simulink model "a20210929KillSwitchCharging"  (R2021b)
settings: Solver=VariableStepAuto  StartTime=0.0  StopTime=inf  RelTol=1e-3
model workspace (MAT data in the model file):
  Ah_chg = [23.2 23.2]
  Ah_dsg = [46.4 46.4]
  R_chg = [0.512  0.512; 0.424  0.424; 0.352  0.352; 0.28  0.28]
  R_dsg = [0.128  0.128; 0.106  0.106; 0.088  0.088; 0.07  0.07]
  T = [298.15 323.15]
  V_chg = [186.88  186.88; 224.64  224.64; 247.68  247.68; 266.88  266.88]
  V_dsg = [93.44  93.44; 112.32  112.32; 123.84  123.84; 133.44  133.44]
  soc = [0 0.25 0.75 1]
libraries: fl_lib x42, nesl_utility x38, ee_lib x19, spsOnDelayLib x1
(part 1 of 2)
settings Model: Creator=phunith  LastModifiedBy=Windows 11

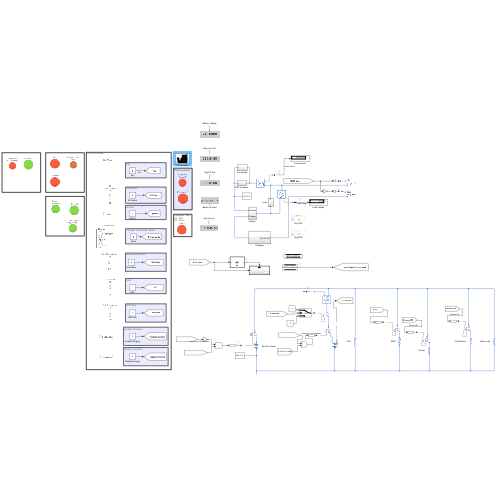
[thumbnail: Simulink's stored preview of the top-level diagram]
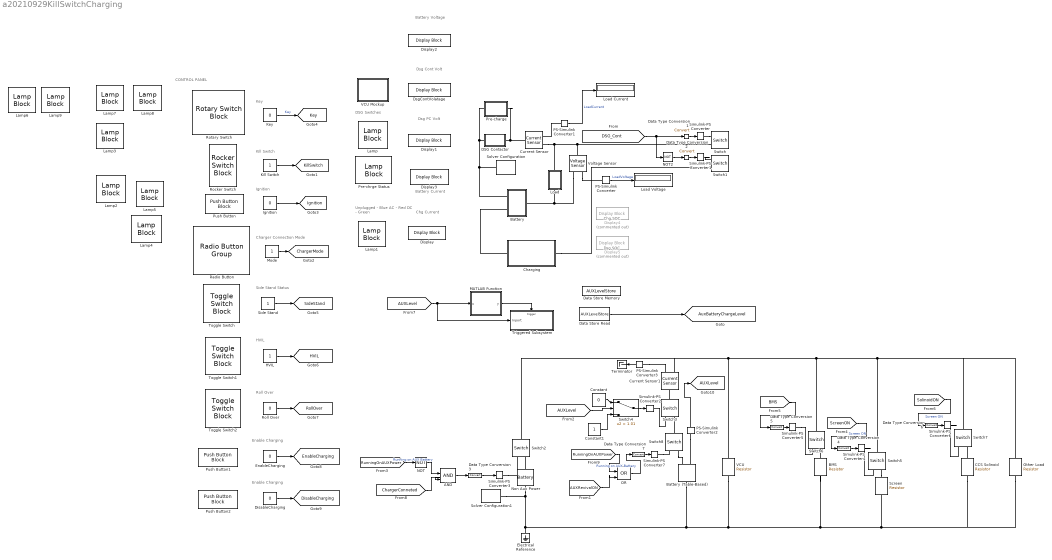
== system a20210929KillSwitchCharging ==
  note: Roll Over
  note: HVIL
  note: Side Stand Status
  note: Key
  note: Charger Connection Mode
  note: Ignition
  note: Kill Switch
  note: Dsg SOC
  note: Chg SOC
  note: DSG Switches
  note: Unplugged - Blue
      | AC - Red
      | DC - Green
  note: Battery Voltage
  note: Dsg PC Volt
  note: Dsg Cont Volt
  note: CONTROL PANEL
  note: Chg Current
  note: Battery Current
  note: Enable Charging
  note: Enable Charging
  AND : Logic  IconShape=distinctive  AllPortsSameDT=off  OutDataTypeStr=boolean
  BMS : fl_lib/Electrical/Electrical Elements/Resistor  R=1 Ohm  i_specify=off  i_priority=None  i=0 A  i_nominal_specify=off  i_nominal_unit=A  i_nominal_value=1  v_specify=off  v_priority=None  v=0 V  v_nominal_specify=off  v_nominal_unit=V  v_nominal_value=1
  Battery : Subsystem
      settings: PortSchema="{\"entries\":[{\"content\":{\"sides\":[{\"content\":{\"connectorIds\":[]},\"type\":\"ConnectorPlacement.EquallySpacedRectSide\",\"uuid\":\"3d16cdf9-dd27-491e-ad4b-7ae493a50ab6\"},{\"content\":{\"connectorIds\":[],\"side\":\"RIGHT\"},\"type\":\"ConnectorPlacement.EquallySpacedRectSide\",\"uuid\":\"1ccab280-74c9-429c-a924-5e281bdde4c9\"},{\"content\":{\"connectorIds\":[\"LConn1\",\"LConn2\"],\"side\":\"TOP\"},\"type\":\"ConnectorPlacement.EquallySpacedRectSide\",\"uuid\":\"a1cee76e-723c-4fd6-b515-6922975a2d3c\"},{\"content\":{\"connectorIds\":[\"RConn1\"],\"side\":\"BOTTOM\"},\"type\":\"ConnectorPlacement.EquallySpacedRectSide\",\"uuid\":\"a5651c44-3216-47cd-a00a-ded9628cada7\"}]},\"type\":\"ConnectorPlacement.EquallySpacedConnector\",\"uuid\":\"8fdcce07-83bd-45b7-89d6-c65ad780a98b\"}],\"packageUris\":[\"http://schema.mathworks.com/mf0/Connector/R2020b\"],\"version\":\"1.0\"}"
  Battery (Table-Based) : ee_lib/Sources/Battery (Table-Based)  SOC_vec=[0, .25, .75, 1]  T_dependence=ee.enum.temperature_dependence.yes  prm_dir=ee.enum.battery.prm_dir.noCurrentDirectionality  T_vec=[273.15, 298.15, 323.15] K  V0_mat=[3.2, 3.1, 3.14; 3.25, 3.27, 3.3; 3.28, 3.31, 3.34; 3.33, 3.5, 3.59] V  V0_vec=[3.1, 3.27, 3.31, 3.5] V  R0_mat=[.03, .015, .002; .04, .017, .008; .039, .012, .006; .027, .013, .021] Ohm  R0_vec=[.015, .017, .012, .013] Ohm  R0_dis_mat=[.03, .015, .002; .04, .017, .008; .039, .012, .006; .027, .013, .021] Ohm  R0_dis_vec=[.015, .017, .012, .013] Ohm  R0_ch_mat=[.03, .015, .002; .04, .017, .008; .039, .012, .006; .027, .013, .021] Ohm  R0_ch_vec=[.015, .017, .012, .013] Ohm  AH_vec=[2.9, 4.1, 4.2] hr*A  AH=4.1 hr*A  prm_leak=ee.enum.battery.prm_leak.disabled  Rleak_vec=[8000, 7000, 6000] Ohm  Rleak=7e3 Ohm  extrapolation_option=ee.enum.extrapolation.nearest  prm_dyn=ee.enum.battery.prm_dyn.off  R1_mat=[.089, .076, .01; .042, .022, .099; .019, .007, .002; .051, .043, .029] Ohm  R1_vec=[.076, .022, .007, .043] Ohm  tau1_mat=[44, 148, 235; 93, 110, 1000; 19, 27, 133; .5, 22, 3] s  tau1_vec=[148, 110, 27, 22] s  R2_mat=[.014, .382, .407; .028, .006, .007; .014, .007, .006; .333, .956, .912] Ohm  R2_vec=[.382, .006, .007, .956] Ohm  tau2_mat=[1, 44, 5644; 11, 24, 506; 2, 14, 330; 3310, 13419, 30216] s  tau2_vec=[44, 24, 14, 13419] s  R3_mat=[.014, .382, .407; .028, .006, .007; .014, .007, .006; .333, .956, .912] Ohm  R3_vec=[.382, .006, .007, .956] Ohm  tau3_mat=[1, 44, 5644; 11, 24, 506; 2, 14, 330; 3310, 13419, 30216] s  tau3_vec=[44, 24, 14, 13419] s  R4_mat=[.014, .382, .407; .028, .006, .007; .014, .007, .006; .333, .956, .912] Ohm  R4_vec=[.382, .006, .007, .956] Ohm  tau4_mat=[1, 44, 5644; 11, 24, 506; 2, 14, 330; 3310, 13419, 30216] s  tau4_vec=[44, 24, 14, 13419] s  R5_mat=[.014, .382, .407; .028, .006, .007; .014, .007, .006; .333, .956, .912] Ohm  R5_vec=[.382, .006, .007, .956] Ohm  tau5_mat=[1, 44, 5644; 11, 24, 506; 2, 14, 330; 3310, 13419, 30216] s  tau5_vec=[44, 24, 14, 13419] s  prm_fade=ee.enum.battery.prm_fade.equations  N0=100  dV0=0  dR0=0  dAH=0  dRleak=0  dR1=0  dR2=0  dR3=0  dR4=0  dR5=0  N0vec=[100, 200, 300]  Tfadevec=[298.15, 323.15] K  dV0vec=[0, 0, 0]  dR0vec=[0, 0, 0]  dAHvec=[0, 0, 0]  dRleakvec=[0, 0, 0]  dR1vec=[0, 0, 0]  dR2vec=[0, 0, 0]  dR3vec=[0, 0, 0]  dR4vec=[0, 0, 0]  dR5vec=[0, 0, 0]  dV0mat=[0, 0; 0, 0; 0, 0]  dR0mat=[0, 0; 0, 0; 0, 0]  dAHmat=[0, 0; 0, 0; 0, 0]  dRleakmat=[0, 0; 0, 0; 0, 0]  dR1mat=[0, 0; 0, 0; 0, 0]  dR2mat=[0, 0; 0, 0; 0, 0]  dR3mat=[0, 0; 0, 0; 0, 0]  dR4mat=[0, 0; 0, 0; 0, 0]  dR5mat=[0, 0; 0, 0; 0, 0]  prm_age=ee.enum.battery.prm_age.disabled  prm_age_OCV=ee.enum.battery.prm_age_OCV.OCV  OCV_age=0.9  SOC_age=0.6  storage_dt_age_vec=[0] d  storage_T_age_vec=[273] K  OCV_scaling_age=2.2134e6  OCV_offset_age=1.632e6  temp_exp_age=0.515833569 V  t_exp_age=0.75  T_age_vec=[273.15, 298.15, 323.15] K  dt_age_vec=[90, 180, 270, 360] d  dR0_age_vec=[0, 0, 0]  t_meas_dR0_age=100 d  dR0_age_mat=[0, 0, 0; 0, 0, 0; 0, 0, 0; 0, 0, 0]  temperature=298.15 K  i_specify=off  i_priority=None  i=0 A  i_nominal_specify=off  i_nominal_unit=A  i_nominal_value=1  v_specify=off  v_priority=None  v=0 V  v_nominal_specify=off  v_nominal_unit=V  v_nominal_value=1  stateOfCharge_specify=off  stateOfCharge_priority=High  stateOfCharge=1  stateOfCharge_nominal_specify=off  stateOfCharge_nominal_unit=1  stateOfCharge_nominal_value=1  num_cycles_specify=off  num_cycles_priority=High  num_cycles=0  num_cycles_nominal_specify=off  num_cycles_nominal_unit=1  num_cycles_nominal_value=1  thermal_mass=30000 J/K  temperature_specify=off  temperature_priority=High  temperature_nominal_specify=off  temperature_nominal_unit=K  temperature_nominal_value=1
      settings: SourceProductBaseCode=PS  InternalSimscapePortConfiguration="{\"Bottom\":[],\"Left\":[{\"id\":\"p\",\"label\":\"+\",\"type\":\"foundation.electrical.electrical\"},{\"id\":\"soc\",\"label\":\"SOC\",\"type\":\"output\"}],\"Right\":[{\"id\":\"n\",\"label\":\"-\",\"type\":\"foundation.electrical.electrical\"}],\"Top\":[]}"
  CCS Solinoid : fl_lib/Electrical/Electrical Elements/Resistor  R=1 Ohm  i_specify=off  i_priority=None  i=0 A  i_nominal_specify=off  i_nominal_unit=A  i_nominal_value=1  v_specify=off  v_priority=None  v=0 V  v_nominal_specify=off  v_nominal_unit=V  v_nominal_value=1
  Charging : Subsystem
  Constant : Constant  Value=0
  Constant1 : Constant
  Current Sensor : fl_lib/Electrical/Electrical Sensors/Current Sensor
  Current Sensor1 : fl_lib/Electrical/Electrical Sensors/Current Sensor
  DSG Contactor : Subsystem
  Data Store Memory : DataStoreMemory  DataStoreName=AUXLevelStore  ReadBeforeWriteMsg=warning  WriteAfterWriteMsg=warning  WriteAfterReadMsg=warning  InitialValue=1  ShowAdditionalParam=off
  Data Store Read : DataStoreRead  DataStoreName=AUXLevelStore  IndexOptions=Index vector (dialog)  Indices=1  OutputSizes=1
  Data Type Conversion{1..7} (7 alike) : DataTypeConversion
  DisableCharging : Constant  Value=0
  Display{,1..3} (4 alike) : DisplayBlock  LabelPosition=Hide  Format=short  Transparency=1
  Display4 : DisplayBlock  Commented=on  LabelPosition=Hide  Format=short  Transparency=1
  Display5 : DisplayBlock  Commented=on  LabelPosition=Hide  Format=short  Transparency=1
  DsgContVolatage : DisplayBlock  LabelPosition=Hide  Format=short  Transparency=1
  Electrical Reference : fl_lib/Electrical/Electrical Elements/Electrical Reference
  EnableCharging : Constant  Value=0
  HVIL : Constant
  Ignition : Constant  Value=0
  Key : Constant  Value=0
  Kill Switch : Constant
  Lamp{,1..9} (10 alike) : LampBlock
  Load : Subsystem
  Load Current : Display
  Load Voltage : Display
  MATLAB Function : MATLAB Function  TreatAsAtomicUnit=on
  Mode : Constant
  NOT : Logic  Operator=NOT  IconShape=distinctive  AllPortsSameDT=off  OutDataTypeStr=boolean
  NOT2 : Logic  Operator=NOT  IconShape=distinctive  AllPortsSameDT=off  OutDataTypeStr=boolean
  Non Aux Power : ee_lib/Sources/Battery  Vnom=120 V  prm_dir=1  R1_dis=2 Ohm  R1_ch=2 Ohm  R1=1 Ohm  prm_AH=1  AH=50 hr*A  V1=11.5 V  AH1=25 hr*A  prm_R2=1  R2=2000 Ohm  prm_dyn=1  Rp1=0.005 Ohm  tau1=30 s  Rp2=0.005 Ohm  tau2=30 s  Rp3=0.005 Ohm  tau3=30 s  Rp4=0.005 Ohm  tau4=30 s  Rp5=0.005 Ohm  tau5=30 s  prm_fade=1  N_fade=100  AH_fade=45 hr*A  R1_fade=2.02 Ohm  R1_ch_fade=2.02 Ohm  V1_fade=10.35 V  prm_age=1  prm_age_OCV=1  OCV_age=0.9  SOC_age=60  delta_time_age_vec=[0] d  temperature_age_vec=[273] K  OCV_scaling_age=2.2134e6  OCV_offset_age=1.632e6  temp_exp_age=0.515833569 V  t_exp_age=0.75  i_specify=off  i_priority=None  i=0 A  i_nominal_specify=off  i_nominal_unit=A  i_nominal_value=1  v_specify=off  v_priority=None  v=0 V  v_nominal_specify=off  v_nominal_unit=V  v_nominal_value=1  charge_specify=off  charge_priority=High  charge=50 hr*A  charge_nominal_specify=off  charge_nominal_unit=hr*A  charge_nominal_value=1  num_cycles_specify=off  num_cycles_priority=High  num_cycles=0  num_cycles_nominal_specify=off  num_cycles_nominal_unit=1  num_cycles_nominal_value=1  Tmeas=298.15 K  Tmeas_age=298.15 K  Vnom_T2=12 V  R1_T2=2.2 Ohm  R1_T2_dis=2.2 Ohm  R1_T2_ch=2.2 Ohm  V1_T2=11.4 V  R2_T2=2200 Ohm  Rp1_T2=0.005 Ohm  tau1_T2=30 s  Rp2_T2=0.005 Ohm  tau2_T2=30 s  Rp3_T2=0.005 Ohm  tau3_T2=30 s  Rp4_T2=0.005 Ohm  tau4_T2=30 s  Rp5_T2=0.005 Ohm  tau5_T2=30 s  Tmeas2=273.15 K  thermal_mass=30000 J/K  temperature_specify=off  temperature_priority=High  temperature=298.15 K  temperature_nominal_specify=off  temperature_nominal_unit=K  temperature_nominal_value=1
  OR : Logic  Operator=OR  IconShape=distinctive  AllPortsSameDT=off  OutDataTypeStr=boolean
  Other Load : fl_lib/Electrical/Electrical Elements/Resistor  R=10 Ohm  i_specify=off  i_priority=None  i=0 A  i_nominal_specify=off  i_nominal_unit=A  i_nominal_value=1  v_specify=off  v_priority=None  v=0 V  v_nominal_specify=off  v_nominal_unit=V  v_nominal_value=1
  PS-Simulink Converter{,1..3} (4 alike) : nesl_utility/PS-Simulink Converter  PhysicalDomain=network_engine_domain  SubClassName=ps_output  LeftPortType=input  RightPortType=output  PseudoPeriodic=off  Frequencies=[]  Unit=inherit  AffineConversion=off
      settings: SourceProductBaseCode=PW,SS
  Pre-charge : Subsystem
  Pre-chrge Status : LampBlock
  Push Button : PushButtonBlock  ButtonText=Ignition  OffValue=0.000000
  Push Button1 : PushButtonBlock  ButtonText=Enable Charging  OffValue=0.000000
  Push Button2 : PushButtonBlock  ButtonText=Disable Charging  OffValue=0.000000
  Radio Button : RadioButtonGroup  SelectedLabel=AC  ButtonGroupName=Charger
      settings: Values={{'Unplugged', 'AC', 'DC'}, [0 1 2]}
  Rocker Switch : RockerSwitchBlock
      settings: Values={{'Off', 'On'}, [0 1]}
  Roll Over : Constant  Value=0
  Rotary Switch : RotarySwitchBlock
      settings: Values={{'Off', 'On'}, [0 1]}
  Screen : fl_lib/Electrical/Electrical Elements/Resistor  R=1 Ohm  i_specify=off  i_priority=None  i=0 A  i_nominal_specify=off  i_nominal_unit=A  i_nominal_value=1  v_specify=off  v_priority=None  v=0 V  v_nominal_specify=off  v_nominal_unit=V  v_nominal_value=1
  Side Stand : Constant
  Simulink-PS Converter{,1..7} (8 alike) : nesl_utility/Simulink-PS Converter  PhysicalDomain=network_engine_domain  SubClassName=ps_input  LeftPortType=input  RightPortType=output  PseudoPeriodic=off  Frequencies=[]  NoiseDistribution=none  NoiseParameters=[]  Unit=1  AffineConversion=off  FilteringAndDerivatives=provide  SimscapeFilterOrder=1  InputFilterTimeConstant=0.001  UdotUserProvided=0
      settings: SourceProductBaseCode=PW,SS
  Solver Configuration : nesl_utility/Solver Configuration  PhysicalDomain=network_engine_domain  SubClassName=solver  LeftPortType=input  RightPortType=generic  Tones=[]  Harmonics=[]  SimulateNoise=off  Profile=off  UseLocalSampling=off  EnableSwitchedLinearOptims=on  FrequencyDomain=off  UseCCode=off  RelTol=0.001  AbsTol=1e-06  MinStep=1e-09  ToWorkspace=off  RevertToSquareIcSolve=off  NumHomotopyIterations=100  PhasorMode=off  PhasorModeNumHarmonics=1  DoDC=off  ResidualTolerance=1e-09  UseLocalSolver=off  LocalSolverChoice=NE_BACKWARD_EULER_ADVANCER  LocalSolverSampleTime=0.001  DoFixedCost=off  MaxNonlinIter=3  MaxModeIter=2  ComputeImpulses=off  ImpulseIterations=2  LinearAlgebra=auto  EquationFormulation=NE_TIME_EF  DelaysMemoryBudget=1024  AutomaticFiltering=on  FilteringTimeConstant=0.001  PartitionStorageMethod=AS_NEEDED  PartitionMemoryBudget=1024  PartitionMethod=ROBUST
      settings: SourceProductBaseCode=PW,SS
  Solver Configuration1 : nesl_utility/Solver Configuration  PhysicalDomain=network_engine_domain  SubClassName=solver  LeftPortType=input  RightPortType=generic  Tones=[]  Harmonics=[]  SimulateNoise=off  Profile=off  UseLocalSampling=off  EnableSwitchedLinearOptims=on  FrequencyDomain=off  UseCCode=off  RelTol=0.001  AbsTol=1e-06  MinStep=1e-09  ToWorkspace=off  RevertToSquareIcSolve=off  NumHomotopyIterations=100  PhasorMode=off  PhasorModeNumHarmonics=1  DoDC=off  ResidualTolerance=1e-09  UseLocalSolver=off  LocalSolverChoice=NE_BACKWARD_EULER_ADVANCER  LocalSolverSampleTime=0.001  DoFixedCost=off  MaxNonlinIter=3  MaxModeIter=2  ComputeImpulses=off  ImpulseIterations=2  LinearAlgebra=auto  EquationFormulation=NE_TIME_EF  DelaysMemoryBudget=1024  AutomaticFiltering=on  FilteringTimeConstant=0.001  PartitionStorageMethod=AS_NEEDED  PartitionMemoryBudget=1024  PartitionMethod=ROBUST
      settings: SourceProductBaseCode=PW,SS
  Switch{,1..3,5..8} (8 alike) : fl_lib/Electrical/Electrical Elements/Switch  R_closed=0.01 Ohm  G_open=1e-8 1/Ohm  Threshold=0.5  i_specify=off  i_priority=None  i=0 A  i_nominal_specify=off  i_nominal_unit=A  i_nominal_value=1  v_specify=off  v_priority=None  v=0 V  v_nominal_specify=off  v_nominal_unit=V  v_nominal_value=1
  Switch4 : Switch  Criteria=u2 > Threshold  Threshold=1.01
  Terminator : Terminator
  Toggle Switch : ToggleSwitchBlock
      settings: Values={{'Off', 'On'}, [0 1]}
  Toggle Switch1 : ToggleSwitchBlock
      settings: Values={{'Off', 'On'}, [0 1]}
  Toggle Switch2 : ToggleSwitchBlock
      settings: Values={{'Off', 'On'}, [0 1]}
  Triggered Subsystem : Subsystem  TreatAsAtomicUnit=on
  VCU : fl_lib/Electrical/Electrical Elements/Resistor  R=10 Ohm  i_specify=off  i_priority=None  i=0 A  i_nominal_specify=off  i_nominal_unit=A  i_nominal_value=1  v_specify=off  v_priority=None  v=0 V  v_nominal_specify=off  v_nominal_unit=V  v_nominal_value=1
  VCU Mockup : Subsystem
  Voltage Sensor : fl_lib/Electrical/Electrical Sensors/Voltage Sensor
  tag scope: AUXLevel=global, AuxBatteryChargeLevel=global, ChargerMode=global, DisableCharging=global, EnableCharging=global, HVIL=global, Ignition=global, Key=global, KillSwitch=global, RollOver=global, SideStand=global
  wires:
  PS-Simulink Converter/1 -> Load Voltage/1  "LoadVoltage"
  PS-Simulink Converter1/1 -> Load Current/1  "LoadCurrent"
  Kill Switch/1 -> [KillSwitch]
  Ignition/1 -> [Ignition]
  Mode/1 -> [ChargerMode]
  Key/1 -> [Key]  "Key"
  Side Stand/1 -> [SideStand]
  HVIL/1 -> [HVIL]
  Roll Over/1 -> [RollOver]
  EnableCharging/1 -> [EnableCharging]
  DisableCharging/1 -> [DisableCharging]
  Data Type Conversion1/1 -> Simulink-PS Converter/1
  Data Type Conversion2/1 -> Simulink-PS Converter1/1
  [DSG_Cont] -> NOT2/1, Data Type Conversion1/1
  Data Type Conversion3/1 -> Simulink-PS Converter3/1
  [RunningOnAUXPower] -> NOT/1  "Running on AUX Battery"
  [AUXLevel] -> Switch4/2
  Constant/1 -> Switch4/1
  Constant1/1 -> Switch4/3
  Switch4/1 -> Simulink-PS Converter2/1
  Data Type Conversion4/1 -> Simulink-PS Converter4/1
  [ScreenON] -> Data Type Conversion4/1  "Screen ON"
  [BMS] -> Data Type Conversion5/1
  Data Type Conversion5/1 -> Simulink-PS Converter5/1
  [SolinoidON] -> Data Type Conversion6/1  "Screen ON"
  Data Type Conversion6/1 -> Simulink-PS Converter6/1
  Data Store Read/1 -> [AuxBatteryChargeLevel]
  MATLAB Function/1(y) -> Triggered Subsystem/Trigger
  [AUXLevel] -> MATLAB Function/1(u), Triggered Subsystem/1(Inport)
  [RunningOnAUXPower] -> OR/1  "Running on AUX Battery"
  Data Type Conversion7/1 -> Simulink-PS Converter7/1
  PS-Simulink Converter3/1 -> Terminator/1
  PS-Simulink Converter2/1 -> [AUXLevel]
  NOT2/1 -> Data Type Conversion2/1
  [AUXRevivalON] -> OR/2
  OR/1 -> Data Type Conversion7/1
  [ChargerConneted] -> AND/2
  NOT/1 -> AND/1
  AND/1 -> Data Type Conversion3/1
  connections:
  Battery/LConn1 -- Pre-charge/LConn1 -- DSG Contactor/LConn1 -- Solver Configuration/RConn1
  Pre-charge/RConn1 -- Current Sensor/LConn1 -- DSG Contactor/RConn1
  Voltage Sensor/RConn2 -- Battery/RConn1 -- Load/RConn1
  Voltage Sensor/RConn1 -- PS-Simulink Converter/LConn1
  Voltage Sensor/LConn1 -- Switch/RConn2 -- Current Sensor/RConn2 -- Load/LConn1
  PS-Simulink Converter1/LConn1 -- Current Sensor/RConn1
  Simulink-PS Converter/RConn1 -- Switch/RConn1
  Charging/RConn1 -- Switch1/RConn2
  Charging/LConn1 -- Battery/LConn2
  Simulink-PS Converter1/RConn1 -- Switch1/RConn1
  Simulink-PS Converter3/RConn1 -- Switch2/RConn1
  PS-Simulink Converter2/LConn1 -- Battery (Table-Based)/LConn2
  VCU/LConn1 -- Current Sensor1/RConn2 -- Switch2/LConn1 -- Switch6/LConn1 -- Switch7/LConn1 -- Other Load/LConn1 -- Switch5/LConn1
  Non Aux Power/RConn1 -- Solver Configuration1/RConn1 -- Electrical Reference/LConn1 -- Battery (Table-Based)/RConn1 -- VCU/RConn1 -- Other Load/RConn1 -- CCS Solinoid/RConn1 -- Screen/RConn1 -- BMS/RConn1
  Non Aux Power/LConn1 -- Switch2/RConn2
  Simulink-PS Converter2/RConn1 -- Switch3/RConn1
  Switch5/RConn2 -- Screen/LConn1
  Simulink-PS Converter4/RConn1 -- Switch5/RConn1
  Simulink-PS Converter5/RConn1 -- Switch6/RConn1
  BMS/LConn1 -- Switch6/RConn2
  Simulink-PS Converter6/RConn1 -- Switch7/RConn1
  CCS Solinoid/LConn1 -- Switch7/RConn2
  Switch8/LConn1 -- Switch3/RConn2
  Switch8/RConn2 -- Battery (Table-Based)/LConn1
  Simulink-PS Converter7/RConn1 -- Switch8/RConn1
  Switch3/LConn1 -- Current Sensor1/LConn1
  PS-Simulink Converter3/LConn1 -- Current Sensor1/RConn1

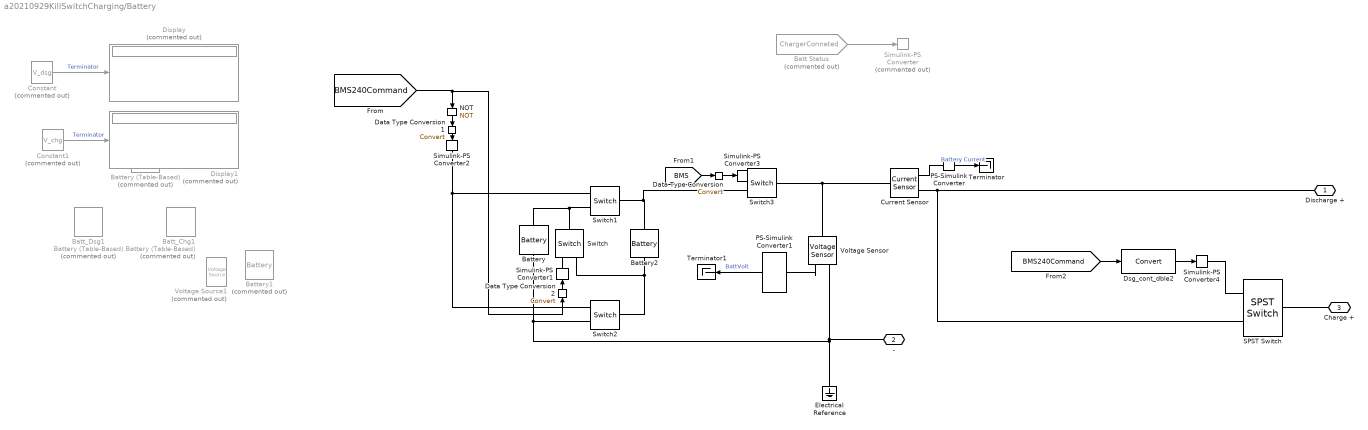
== system a20210929KillSwitchCharging/Battery ==
  Batt Status : From  Commented=on  GotoTag=ChargerConneted  TagVisibility=global
  Batt_Chg1 : ee_lib/Sources/Battery (Table-Based)  Commented=on  SOC_vec=[0 0.25 0.75 1]  T_dependence=ee.enum.temperature_dependence.yes  prm_dir=ee.enum.battery.prm_dir.noCurrentDirectionality  T_vec=[298.15 323.15] K  V0_mat=V_chg V  V0_vec=[3.1, 3.27, 3.31, 3.5] V  R0_mat=[0.512 0.512;0.424 0.424;0.352 0.352;0.28 0.28] Ohm  R0_vec=[.015, .017, .012, .013] Ohm  R0_dis_mat=[.03, .015, .002; .04, .017, .008; .039, .012, .006; .027, .013, .021] Ohm  R0_dis_vec=[.015, .017, .012, .013] Ohm  R0_ch_mat=[.03, .015, .002; .04, .017, .008; .039, .012, .006; .027, .013, .021] Ohm  R0_ch_vec=[.015, .017, .012, .013] Ohm  AH_vec=Ah_chg hr*A  AH=4.1 hr*A  prm_leak=ee.enum.battery.prm_leak.disabled  Rleak_vec=[8000, 7000, 6000] Ohm  Rleak=7e3 Ohm  extrapolation_option=ee.enum.extrapolation.nearest  prm_dyn=ee.enum.battery.prm_dyn.off  R1_mat=[.089, .076, .01; .042, .022, .099; .019, .007, .002; .051, .043, .029] Ohm  R1_vec=[.076, .022, .007, .043] Ohm  tau1_mat=[44, 148, 235; 93, 110, 1000; 19, 27, 133; .5, 22, 3] s  tau1_vec=[148, 110, 27, 22] s  R2_mat=[.014, .382, .407; .028, .006, .007; .014, .007, .006; .333, .956, .912] Ohm  R2_vec=[.382, .006, .007, .956] Ohm  tau2_mat=[1, 44, 5644; 11, 24, 506; 2, 14, 330; 3310, 13419, 30216] s  tau2_vec=[44, 24, 14, 13419] s  R3_mat=[.014, .382, .407; .028, .006, .007; .014, .007, .006; .333, .956, .912] Ohm  R3_vec=[.382, .006, .007, .956] Ohm  tau3_mat=[1, 44, 5644; 11, 24, 506; 2, 14, 330; 3310, 13419, 30216] s  tau3_vec=[44, 24, 14, 13419] s  R4_mat=[.014, .382, .407; .028, .006, .007; .014, .007, .006; .333, .956, .912] Ohm  R4_vec=[.382, .006, .007, .956] Ohm  tau4_mat=[1, 44, 5644; 11, 24, 506; 2, 14, 330; 3310, 13419, 30216] s  tau4_vec=[44, 24, 14, 13419] s  R5_mat=[.014, .382, .407; .028, .006, .007; .014, .007, .006; .333, .956, .912] Ohm  R5_vec=[.382, .006, .007, .956] Ohm  tau5_mat=[1, 44, 5644; 11, 24, 506; 2, 14, 330; 3310, 13419, 30216] s  tau5_vec=[44, 24, 14, 13419] s  prm_fade=ee.enum.battery.prm_fade.equations  N0=100  dV0=0  dR0=0  dAH=0  dRleak=0  dR1=0  dR2=0  dR3=0  dR4=0  dR5=0  N0vec=[100, 200, 300]  Tfadevec=[298.15, 323.15] K  dV0vec=[0, 0, 0]  dR0vec=[0, 0, 0]  dAHvec=[0, 0, 0]  dRleakvec=[0, 0, 0]  dR1vec=[0, 0, 0]  dR2vec=[0, 0, 0]  dR3vec=[0, 0, 0]  dR4vec=[0, 0, 0]  dR5vec=[0, 0, 0]  dV0mat=[0, 0; 0, 0; 0, 0]  dR0mat=[0, 0; 0, 0; 0, 0]  dAHmat=[0, 0; 0, 0; 0, 0]  dRleakmat=[0, 0; 0, 0; 0, 0]  dR1mat=[0, 0; 0, 0; 0, 0]  dR2mat=[0, 0; 0, 0; 0, 0]  dR3mat=[0, 0; 0, 0; 0, 0]  dR4mat=[0, 0; 0, 0; 0, 0]  dR5mat=[0, 0; 0, 0; 0, 0]  prm_age=ee.enum.battery.prm_age.disabled  prm_age_OCV=ee.enum.battery.prm_age_OCV.OCV  OCV_age=0.9  SOC_age=0.6  storage_dt_age_vec=[0] d  storage_T_age_vec=[273] K  OCV_scaling_age=2.2134e6  OCV_offset_age=1.632e6  temp_exp_age=0.515833569 V  t_exp_age=0.75  T_age_vec=[273.15, 298.15, 323.15] K  dt_age_vec=[90, 180, 270, 360] d  dR0_age_vec=[0, 0, 0]  t_meas_dR0_age=100 d  dR0_age_mat=[0, 0, 0; 0, 0, 0; 0, 0, 0; 0, 0, 0]  temperature=298.15 K  i_specify=off  i_priority=None  i=0 A  i_nominal_specify=off  i_nominal_unit=A  i_nominal_value=1  v_specify=off  v_priority=None  v=0 V  v_nominal_specify=off  v_nominal_unit=V  v_nominal_value=1  stateOfCharge_specify=on  stateOfCharge_priority=High  stateOfCharge=0.5  stateOfCharge_nominal_specify=off  stateOfCharge_nominal_unit=1  stateOfCharge_nominal_value=1  num_cycles_specify=off  num_cycles_priority=High  num_cycles=0  num_cycles_nominal_specify=off  num_cycles_nominal_unit=1  num_cycles_nominal_value=1  thermal_mass=30000 J/K  temperature_specify=off  temperature_priority=High  temperature_nominal_specify=off  temperature_nominal_unit=K  temperature_nominal_value=1
      settings: SourceProductBaseCode=PS  InternalSimscapePortConfiguration="{\"Bottom\":[],\"Left\":[{\"id\":\"p\",\"label\":\"+\",\"type\":\"foundation.electrical.electrical\"},{\"id\":\"soc\",\"label\":\"SOC\",\"type\":\"output\"}],\"Right\":[{\"id\":\"n\",\"label\":\"-\",\"type\":\"foundation.electrical.electrical\"}],\"Top\":[]}"
  Batt_Dsg1 : ee_lib/Sources/Battery (Table-Based)  Commented=on  SOC_vec=soc  T_dependence=ee.enum.temperature_dependence.yes  prm_dir=ee.enum.battery.prm_dir.noCurrentDirectionality  T_vec=T K  V0_mat=V_dsg V  V0_vec=[3.1, 3.27, 3.31, 3.5] V  R0_mat=R_dsg Ohm  R0_vec=[.015, .017, .012, .013] Ohm  R0_dis_mat=[.03, .015, .002; .04, .017, .008; .039, .012, .006; .027, .013, .021] Ohm  R0_dis_vec=[.015, .017, .012, .013] Ohm  R0_ch_mat=[.03, .015, .002; .04, .017, .008; .039, .012, .006; .027, .013, .021] Ohm  R0_ch_vec=[.015, .017, .012, .013] Ohm  AH_vec=Ah_dsg hr*A  AH=4.1 hr*A  prm_leak=ee.enum.battery.prm_leak.disabled  Rleak_vec=[8000, 7000, 6000] Ohm  Rleak=7e3 Ohm  extrapolation_option=ee.enum.extrapolation.nearest  prm_dyn=ee.enum.battery.prm_dyn.off  R1_mat=[.089, .076, .01; .042, .022, .099; .019, .007, .002; .051, .043, .029] Ohm  R1_vec=[.076, .022, .007, .043] Ohm  tau1_mat=[44, 148, 235; 93, 110, 1000; 19, 27, 133; .5, 22, 3] s  tau1_vec=[148, 110, 27, 22] s  R2_mat=[.014, .382, .407; .028, .006, .007; .014, .007, .006; .333, .956, .912] Ohm  R2_vec=[.382, .006, .007, .956] Ohm  tau2_mat=[1, 44, 5644; 11, 24, 506; 2, 14, 330; 3310, 13419, 30216] s  tau2_vec=[44, 24, 14, 13419] s  R3_mat=[.014, .382, .407; .028, .006, .007; .014, .007, .006; .333, .956, .912] Ohm  R3_vec=[.382, .006, .007, .956] Ohm  tau3_mat=[1, 44, 5644; 11, 24, 506; 2, 14, 330; 3310, 13419, 30216] s  tau3_vec=[44, 24, 14, 13419] s  R4_mat=[.014, .382, .407; .028, .006, .007; .014, .007, .006; .333, .956, .912] Ohm  R4_vec=[.382, .006, .007, .956] Ohm  tau4_mat=[1, 44, 5644; 11, 24, 506; 2, 14, 330; 3310, 13419, 30216] s  tau4_vec=[44, 24, 14, 13419] s  R5_mat=[.014, .382, .407; .028, .006, .007; .014, .007, .006; .333, .956, .912] Ohm  R5_vec=[.382, .006, .007, .956] Ohm  tau5_mat=[1, 44, 5644; 11, 24, 506; 2, 14, 330; 3310, 13419, 30216] s  tau5_vec=[44, 24, 14, 13419] s  prm_fade=ee.enum.battery.prm_fade.equations  N0=100  dV0=0  dR0=0  dAH=0  dRleak=0  dR1=0  dR2=0  dR3=0  dR4=0  dR5=0  N0vec=[100, 200, 300]  Tfadevec=[298.15, 323.15] K  dV0vec=[0, 0, 0]  dR0vec=[0, 0, 0]  dAHvec=[0, 0, 0]  dRleakvec=[0, 0, 0]  dR1vec=[0, 0, 0]  dR2vec=[0, 0, 0]  dR3vec=[0, 0, 0]  dR4vec=[0, 0, 0]  dR5vec=[0, 0, 0]  dV0mat=[0, 0; 0, 0; 0, 0]  dR0mat=[0, 0; 0, 0; 0, 0]  dAHmat=[0, 0; 0, 0; 0, 0]  dRleakmat=[0, 0; 0, 0; 0, 0]  dR1mat=[0, 0; 0, 0; 0, 0]  dR2mat=[0, 0; 0, 0; 0, 0]  dR3mat=[0, 0; 0, 0; 0, 0]  dR4mat=[0, 0; 0, 0; 0, 0]  dR5mat=[0, 0; 0, 0; 0, 0]  prm_age=ee.enum.battery.prm_age.disabled  prm_age_OCV=ee.enum.battery.prm_age_OCV.OCV  OCV_age=0.9  SOC_age=0.6  storage_dt_age_vec=[0] d  storage_T_age_vec=[273] K  OCV_scaling_age=2.2134e6  OCV_offset_age=1.632e6  temp_exp_age=0.515833569 V  t_exp_age=0.75  T_age_vec=[273.15, 298.15, 323.15] K  dt_age_vec=[90, 180, 270, 360] d  dR0_age_vec=[0, 0, 0]  t_meas_dR0_age=100 d  dR0_age_mat=[0, 0, 0; 0, 0, 0; 0, 0, 0; 0, 0, 0]  temperature=298.15 K  i_specify=off  i_priority=None  i=0 A  i_nominal_specify=off  i_nominal_unit=A  i_nominal_value=1  v_specify=off  v_priority=None  v=0 V  v_nominal_specify=off  v_nominal_unit=V  v_nominal_value=1  stateOfCharge_specify=on  stateOfCharge_priority=High  stateOfCharge=1  stateOfCharge_nominal_specify=off  stateOfCharge_nominal_unit=1  stateOfCharge_nominal_value=1  num_cycles_specify=off  num_cycles_priority=High  num_cycles=0  num_cycles_nominal_specify=off  num_cycles_nominal_unit=1  num_cycles_nominal_value=1  thermal_mass=30000 J/K  temperature_specify=off  temperature_priority=High  temperature_nominal_specify=off  temperature_nominal_unit=K  temperature_nominal_value=1
      settings: SourceProductBaseCode=PS  InternalSimscapePortConfiguration="{\"Bottom\":[],\"Left\":[{\"id\":\"p\",\"label\":\"+\",\"type\":\"foundation.electrical.electrical\"},{\"id\":\"soc\",\"label\":\"SOC\",\"type\":\"output\"}],\"Right\":[{\"id\":\"n\",\"label\":\"-\",\"type\":\"foundation.electrical.electrical\"}],\"Top\":[]}"
  Battery : ee_lib/Sources/Battery  Vnom=120 V  prm_dir=1  R1_dis=2 Ohm  R1_ch=2 Ohm  R1=.1 Ohm  prm_AH=2  AH=50 hr*A  V1=11.5 V  AH1=25 hr*A  prm_R2=1  R2=2000 Ohm  prm_dyn=1  Rp1=0.005 Ohm  tau1=30 s  Rp2=0.005 Ohm  tau2=30 s  Rp3=0.005 Ohm  tau3=30 s  Rp4=0.005 Ohm  tau4=30 s  Rp5=0.005 Ohm  tau5=30 s  prm_fade=1  N_fade=100  AH_fade=45 hr*A  R1_fade=2.02 Ohm  R1_ch_fade=2.02 Ohm  V1_fade=10.35 V  prm_age=1  prm_age_OCV=1  OCV_age=0.9  SOC_age=60  delta_time_age_vec=[0] d  temperature_age_vec=[273] K  OCV_scaling_age=2.2134e6  OCV_offset_age=1.632e6  temp_exp_age=0.515833569 V  t_exp_age=0.75  i_specify=off  i_priority=None  i=0 A  i_nominal_specify=off  i_nominal_unit=A  i_nominal_value=1  v_specify=off  v_priority=None  v=0 V  v_nominal_specify=off  v_nominal_unit=V  v_nominal_value=1  charge_specify=off  charge_priority=High  charge=50 hr*A  charge_nominal_specify=off  charge_nominal_unit=hr*A  charge_nominal_value=1  num_cycles_specify=off  num_cycles_priority=High  num_cycles=0  num_cycles_nominal_specify=off  num_cycles_nominal_unit=1  num_cycles_nominal_value=1  Tmeas=298.15 K  Tmeas_age=298.15 K  Vnom_T2=12 V  R1_T2=2.2 Ohm  R1_T2_dis=2.2 Ohm  R1_T2_ch=2.2 Ohm  V1_T2=11.4 V  R2_T2=2200 Ohm  Rp1_T2=0.005 Ohm  tau1_T2=30 s  Rp2_T2=0.005 Ohm  tau2_T2=30 s  Rp3_T2=0.005 Ohm  tau3_T2=30 s  Rp4_T2=0.005 Ohm  tau4_T2=30 s  Rp5_T2=0.005 Ohm  tau5_T2=30 s  Tmeas2=273.15 K  thermal_mass=30000 J/K  temperature_specify=off  temperature_priority=High  temperature=298.15 K  temperature_nominal_specify=off  temperature_nominal_unit=K  temperature_nominal_value=1
  Battery (Table-Based) : ee_lib/Sources/Battery (Table-Based)  Commented=on  SOC_vec=[0, .25, .75, 1]  T_dependence=ee.enum.temperature_dependence.yes  prm_dir=ee.enum.battery.prm_dir.noCurrentDirectionality  T_vec=[273.15, 298.15, 323.15] K  V0_mat=[3.2, 3.1, 3.14; 3.25, 3.27, 3.3; 3.28, 3.31, 3.34; 3.33, 3.5, 3.59] V  V0_vec=[3.1, 3.27, 3.31, 3.5] V  R0_mat=[.03, .015, .002; .04, .017, .008; .039, .012, .006; .027, .013, .021] Ohm  R0_vec=[.015, .017, .012, .013] Ohm  R0_dis_mat=[.03, .015, .002; .04, .017, .008; .039, .012, .006; .027, .013, .021] Ohm  R0_dis_vec=[.015, .017, .012, .013] Ohm  R0_ch_mat=[.03, .015, .002; .04, .017, .008; .039, .012, .006; .027, .013, .021] Ohm  R0_ch_vec=[.015, .017, .012, .013] Ohm  AH_vec=[2.9, 4.1, 4.2] hr*A  AH=4.1 hr*A  prm_leak=ee.enum.battery.prm_leak.disabled  Rleak_vec=[8000, 7000, 6000] Ohm  Rleak=7e3 Ohm  extrapolation_option=ee.enum.extrapolation.nearest  prm_dyn=ee.enum.battery.prm_dyn.off  R1_mat=[.089, .076, .01; .042, .022, .099; .019, .007, .002; .051, .043, .029] Ohm  R1_vec=[.076, .022, .007, .043] Ohm  tau1_mat=[44, 148, 235; 93, 110, 1000; 19, 27, 133; .5, 22, 3] s  tau1_vec=[148, 110, 27, 22] s  R2_mat=[.014, .382, .407; .028, .006, .007; .014, .007, .006; .333, .956, .912] Ohm  R2_vec=[.382, .006, .007, .956] Ohm  tau2_mat=[1, 44, 5644; 11, 24, 506; 2, 14, 330; 3310, 13419, 30216] s  tau2_vec=[44, 24, 14, 13419] s  R3_mat=[.014, .382, .407; .028, .006, .007; .014, .007, .006; .333, .956, .912] Ohm  R3_vec=[.382, .006, .007, .956] Ohm  tau3_mat=[1, 44, 5644; 11, 24, 506; 2, 14, 330; 3310, 13419, 30216] s  tau3_vec=[44, 24, 14, 13419] s  R4_mat=[.014, .382, .407; .028, .006, .007; .014, .007, .006; .333, .956, .912] Ohm  R4_vec=[.382, .006, .007, .956] Ohm  tau4_mat=[1, 44, 5644; 11, 24, 506; 2, 14, 330; 3310, 13419, 30216] s  tau4_vec=[44, 24, 14, 13419] s  R5_mat=[.014, .382, .407; .028, .006, .007; .014, .007, .006; .333, .956, .912] Ohm  R5_vec=[.382, .006, .007, .956] Ohm  tau5_mat=[1, 44, 5644; 11, 24, 506; 2, 14, 330; 3310, 13419, 30216] s  tau5_vec=[44, 24, 14, 13419] s  prm_fade=ee.enum.battery.prm_fade.equations  N0=100  dV0=0  dR0=0  dAH=0  dRleak=0  dR1=0  dR2=0  dR3=0  dR4=0  dR5=0  N0vec=[100, 200, 300]  Tfadevec=[298.15, 323.15] K  dV0vec=[0, 0, 0]  dR0vec=[0, 0, 0]  dAHvec=[0, 0, 0]  dRleakvec=[0, 0, 0]  dR1vec=[0, 0, 0]  dR2vec=[0, 0, 0]  dR3vec=[0, 0, 0]  dR4vec=[0, 0, 0]  dR5vec=[0, 0, 0]  dV0mat=[0, 0; 0, 0; 0, 0]  dR0mat=[0, 0; 0, 0; 0, 0]  dAHmat=[0, 0; 0, 0; 0, 0]  dRleakmat=[0, 0; 0, 0; 0, 0]  dR1mat=[0, 0; 0, 0; 0, 0]  dR2mat=[0, 0; 0, 0; 0, 0]  dR3mat=[0, 0; 0, 0; 0, 0]  dR4mat=[0, 0; 0, 0; 0, 0]  dR5mat=[0, 0; 0, 0; 0, 0]  prm_age=ee.enum.battery.prm_age.disabled  prm_age_OCV=ee.enum.battery.prm_age_OCV.OCV  OCV_age=0.9  SOC_age=0.6  storage_dt_age_vec=[0] d  storage_T_age_vec=[273] K  OCV_scaling_age=2.2134e6  OCV_offset_age=1.632e6  temp_exp_age=0.515833569 V  t_exp_age=0.75  T_age_vec=[273.15, 298.15, 323.15] K  dt_age_vec=[90, 180, 270, 360] d  dR0_age_vec=[0, 0, 0]  t_meas_dR0_age=100 d  dR0_age_mat=[0, 0, 0; 0, 0, 0; 0, 0, 0; 0, 0, 0]  temperature=298.15 K  i_specify=off  i_priority=None  i=0 A  i_nominal_specify=off  i_nominal_unit=A  i_nominal_value=1  v_specify=off  v_priority=None  v=0 V  v_nominal_specify=off  v_nominal_unit=V  v_nominal_value=1  stateOfCharge_specify=off  stateOfCharge_priority=High  stateOfCharge=1  stateOfCharge_nominal_specify=off  stateOfCharge_nominal_unit=1  stateOfCharge_nominal_value=1  num_cycles_specify=off  num_cycles_priority=High  num_cycles=0  num_cycles_nominal_specify=off  num_cycles_nominal_unit=1  num_cycles_nominal_value=1  thermal_mass=30000 J/K  temperature_specify=off  temperature_priority=High  temperature_nominal_specify=off  temperature_nominal_unit=K  temperature_nominal_value=1
      settings: SourceProductBaseCode=PS  InternalSimscapePortConfiguration="{\"Bottom\":[],\"Left\":[{\"id\":\"p\",\"label\":\"+\",\"type\":\"foundation.electrical.electrical\"}],\"Right\":[{\"id\":\"n\",\"label\":\"-\",\"type\":\"foundation.electrical.electrical\"}],\"Top\":[]}"
  Battery1 : ee_lib/Sources/Battery  Commented=on  Vnom=236.8 V  prm_dir=1  R1_dis=2 Ohm  R1_ch=2 Ohm  R1=0.08 Ohm  prm_AH=2  AH=23.2 hr*A  V1=270 V  AH1=12 hr*A  prm_R2=1  R2=2000 Ohm  prm_dyn=1  Rp1=0.005 Ohm  tau1=30 s  Rp2=0.005 Ohm  tau2=30 s  Rp3=0.005 Ohm  tau3=30 s  Rp4=0.005 Ohm  tau4=30 s  Rp5=0.005 Ohm  tau5=30 s  prm_fade=1  N_fade=100  AH_fade=45 hr*A  R1_fade=2.02 Ohm  R1_ch_fade=2.02 Ohm  V1_fade=10.35 V  prm_age=1  prm_age_OCV=1  OCV_age=0.9  SOC_age=60  delta_time_age_vec=[0] d  temperature_age_vec=[273] K  OCV_scaling_age=2.2134e6  OCV_offset_age=1.632e6  temp_exp_age=0.515833569 V  t_exp_age=0.75  i_specify=off  i_priority=None  i=0 A  i_nominal_specify=off  i_nominal_unit=A  i_nominal_value=1  v_specify=off  v_priority=None  v=0 V  v_nominal_specify=off  v_nominal_unit=V  v_nominal_value=1  charge_specify=off  charge_priority=High  charge=50 hr*A  charge_nominal_specify=off  charge_nominal_unit=hr*A  charge_nominal_value=1  num_cycles_specify=off  num_cycles_priority=High  num_cycles=0  num_cycles_nominal_specify=off  num_cycles_nominal_unit=1  num_cycles_nominal_value=1  Tmeas=298.15 K  Tmeas_age=298.15 K  Vnom_T2=12 V  R1_T2=2.2 Ohm  R1_T2_dis=2.2 Ohm  R1_T2_ch=2.2 Ohm  V1_T2=11.4 V  R2_T2=2200 Ohm  Rp1_T2=0.005 Ohm  tau1_T2=30 s  Rp2_T2=0.005 Ohm  tau2_T2=30 s  Rp3_T2=0.005 Ohm  tau3_T2=30 s  Rp4_T2=0.005 Ohm  tau4_T2=30 s  Rp5_T2=0.005 Ohm  tau5_T2=30 s  Tmeas2=273.15 K  thermal_mass=30000 J/K  temperature_specify=off  temperature_priority=High  temperature=298.15 K  temperature_nominal_specify=off  temperature_nominal_unit=K  temperature_nominal_value=1
  Battery2 : ee_lib/Sources/Battery  Vnom=120 V  prm_dir=1  R1_dis=2 Ohm  R1_ch=2 Ohm  R1=.1 Ohm  prm_AH=2  AH=50 hr*A  V1=11.5 V  AH1=25 hr*A  prm_R2=1  R2=2000 Ohm  prm_dyn=1  Rp1=0.005 Ohm  tau1=30 s  Rp2=0.005 Ohm  tau2=30 s  Rp3=0.005 Ohm  tau3=30 s  Rp4=0.005 Ohm  tau4=30 s  Rp5=0.005 Ohm  tau5=30 s  prm_fade=1  N_fade=100  AH_fade=45 hr*A  R1_fade=2.02 Ohm  R1_ch_fade=2.02 Ohm  V1_fade=10.35 V  prm_age=1  prm_age_OCV=1  OCV_age=0.9  SOC_age=60  delta_time_age_vec=[0] d  temperature_age_vec=[273] K  OCV_scaling_age=2.2134e6  OCV_offset_age=1.632e6  temp_exp_age=0.515833569 V  t_exp_age=0.75  i_specify=off  i_priority=None  i=0 A  i_nominal_specify=off  i_nominal_unit=A  i_nominal_value=1  v_specify=off  v_priority=None  v=0 V  v_nominal_specify=off  v_nominal_unit=V  v_nominal_value=1  charge_specify=off  charge_priority=High  charge=50 hr*A  charge_nominal_specify=off  charge_nominal_unit=hr*A  charge_nominal_value=1  num_cycles_specify=off  num_cycles_priority=High  num_cycles=0  num_cycles_nominal_specify=off  num_cycles_nominal_unit=1  num_cycles_nominal_value=1  Tmeas=298.15 K  Tmeas_age=298.15 K  Vnom_T2=12 V  R1_T2=2.2 Ohm  R1_T2_dis=2.2 Ohm  R1_T2_ch=2.2 Ohm  V1_T2=11.4 V  R2_T2=2200 Ohm  Rp1_T2=0.005 Ohm  tau1_T2=30 s  Rp2_T2=0.005 Ohm  tau2_T2=30 s  Rp3_T2=0.005 Ohm  tau3_T2=30 s  Rp4_T2=0.005 Ohm  tau4_T2=30 s  Rp5_T2=0.005 Ohm  tau5_T2=30 s  Tmeas2=273.15 K  thermal_mass=30000 J/K  temperature_specify=off  temperature_priority=High  temperature=298.15 K  temperature_nominal_specify=off  temperature_nominal_unit=K  temperature_nominal_value=1
  Constant : Constant  Commented=on  Value=V_dsg
  Constant1 : Constant  Commented=on  Value=V_chg
  Current Sensor : fl_lib/Electrical/Electrical Sensors/Current Sensor
  Data Type Conversion : DataTypeConversion
  Data Type Conversion1 : DataTypeConversion
  Data Type Conversion2 : DataTypeConversion
  Display : Display  Commented=on
  Display1 : Display  Commented=on
  Dsg_cont_dble2 : DataTypeConversion
  Electrical Reference : fl_lib/Electrical/Electrical Elements/Electrical Reference
  NOT : Logic  Operator=NOT  IconShape=distinctive  AllPortsSameDT=off  OutDataTypeStr=boolean
  PS-Simulink Converter : nesl_utility/PS-Simulink Converter  PhysicalDomain=network_engine_domain  SubClassName=ps_output  LeftPortType=input  RightPortType=output  PseudoPeriodic=off  Frequencies=[]  Unit=inherit  AffineConversion=off
      settings: SourceProductBaseCode=PW,SS
  PS-Simulink Converter1 : nesl_utility/PS-Simulink Converter  PhysicalDomain=network_engine_domain  SubClassName=ps_output  LeftPortType=input  RightPortType=output  PseudoPeriodic=off  Frequencies=[]  Unit=inherit  AffineConversion=off
      settings: SourceProductBaseCode=PW,SS
  SPST Switch : ee_lib/Switches & Breakers/SPST Switch  R_closed=0.01 Ohm  G_open=1e-6 S  Threshold=0.5 V  Width=0 V  model_dynamics=0  t_on=1e-3 s  t_off=1e-3 s  initial_vT=0 V
      settings: SourceProductBaseCode=PS  InternalSimscapePortConfiguration="{\"Bottom\":[],\"Left\":[{\"id\":\"vT\",\"label\":\"vT\",\"type\":\"input\"},{\"id\":\"p\",\"label\":\"\",\"type\":\"foundation.electrical.electrical\"}],\"Right\":[{\"id\":\"n\",\"label\":\"\",\"type\":\"foundation.electrical.electrical\"}],\"Top\":[]}"
  Simulink-PS Converter : nesl_utility/Simulink-PS Converter  Commented=on  PhysicalDomain=network_engine_domain  SubClassName=ps_input  LeftPortType=input  RightPortType=output  PseudoPeriodic=off  Frequencies=[]  NoiseDistribution=none  NoiseParameters=[]  Unit=1  AffineConversion=off  FilteringAndDerivatives=provide  SimscapeFilterOrder=1  InputFilterTimeConstant=0.001  UdotUserProvided=0
      settings: SourceProductBaseCode=PW,SS
  Simulink-PS Converter{1..4} (4 alike) : nesl_utility/Simulink-PS Converter  PhysicalDomain=network_engine_domain  SubClassName=ps_input  LeftPortType=input  RightPortType=output  PseudoPeriodic=off  Frequencies=[]  NoiseDistribution=none  NoiseParameters=[]  Unit=1  AffineConversion=off  FilteringAndDerivatives=provide  SimscapeFilterOrder=1  InputFilterTimeConstant=0.001  UdotUserProvided=0
      settings: SourceProductBaseCode=PW,SS
  Switch{,1..3} (4 alike) : fl_lib/Electrical/Electrical Elements/Switch  R_closed=0.01 Ohm  G_open=1e-8 1/Ohm  Threshold=0.5  i_specify=off  i_priority=None  i=0 A  i_nominal_specify=off  i_nominal_unit=A  i_nominal_value=1  v_specify=off  v_priority=None  v=0 V  v_nominal_specify=off  v_nominal_unit=V  v_nominal_value=1
  Terminator : Terminator
  Terminator1 : Terminator
  Voltage Sensor : fl_lib/Electrical/Electrical Sensors/Voltage Sensor
  Voltage Source1 : ee_lib/Sources/Voltage Source  Commented=on  dc_voltage=120 V  ac_voltage=0 V  ac_shift=0 rad  ac_frequency=60 Hz  noise_mode=0  PSD=0 V^2/Hz  repeatability=1  auto_seed=3499211588  user_seed=0  sample_time=1e-3 s  i_specify=off  i_priority=None  i=0 A  i_nominal_specify=off  i_nominal_unit=A  i_nominal_value=1  v_specify=off  v_priority=None  v=0 V  v_nominal_specify=off  v_nominal_unit=V  v_nominal_value=1
  Discharge + : PMIOPort  Side=Left
  - : PMIOPort  Port=2  Side=Right
  Charge + : PMIOPort  Port=3  Side=Left
  wires:
  PS-Simulink Converter1/1 -> Terminator1/1  "BattVolt"
  Batt Status/1 -> Simulink-PS Converter/1
  Constant/1 -> Display/1  "Terminator"
  Constant1/1 -> Display1/1  "Terminator"
  [BMS240Command] -> Data Type Conversion2/1, NOT/1
  [BMS] -> Data Type Conversion/1
  Data Type Conversion/1 -> Simulink-PS Converter3/1
  NOT/1 -> Data Type Conversion1/1
  Data Type Conversion1/1 -> Simulink-PS Converter2/1
  Data Type Conversion2/1 -> Simulink-PS Converter1/1
  PS-Simulink Converter/1 -> Terminator/1  "Battery Current"
  [BMS240Command] -> Dsg_cont_dble2/1
  Dsg_cont_dble2/1 -> Simulink-PS Converter4/1
  connections:
  Voltage Sensor/RConn1 -- PS-Simulink Converter1/LConn1
  Battery/LConn1 -- Switch/LConn1 -- Switch1/RConn2
  Voltage Sensor/LConn1 -- Current Sensor/LConn1 -- Switch3/LConn1
  Battery2/RConn1 -- Switch/RConn2 -- Switch2/LConn1
  -/RConn1 -- Electrical Reference/LConn1 -- Battery/RConn1 -- Switch2/RConn2 -- Voltage Sensor/RConn2
  Simulink-PS Converter2/RConn1 -- Switch1/RConn1 -- Switch2/RConn1
  Switch1/LConn1 -- Switch3/RConn2 -- Battery2/LConn1
  Simulink-PS Converter3/RConn1 -- Switch3/RConn1
  Simulink-PS Converter1/RConn1 -- Switch/RConn1
  Current Sensor/RConn2 -- SPST Switch/LConn2 -- Discharge +/RConn1
  PS-Simulink Converter/LConn1 -- Current Sensor/RConn1
  Simulink-PS Converter4/RConn1 -- SPST Switch/LConn1
  Charge +/RConn1 -- SPST Switch/RConn1

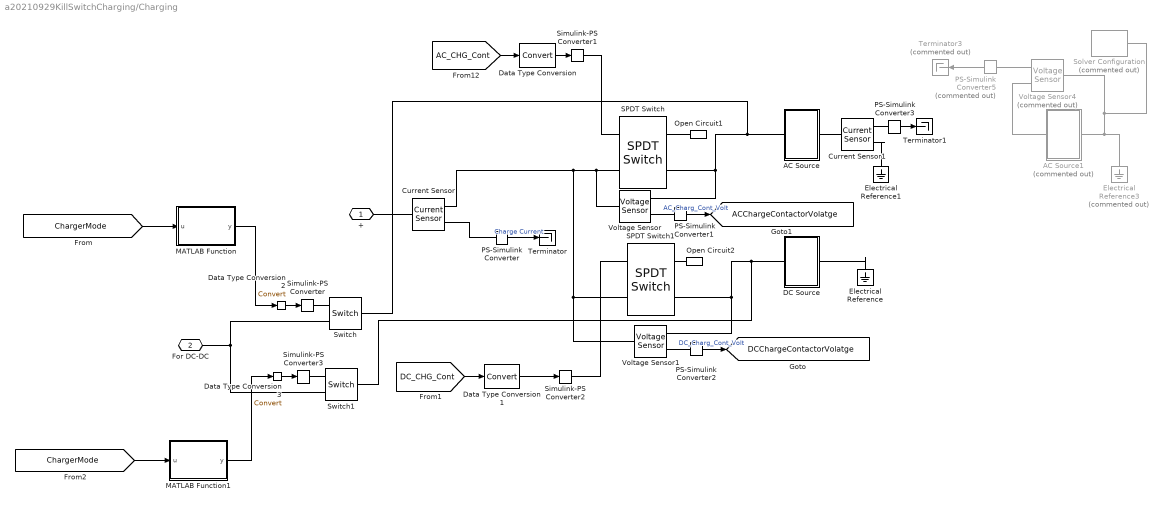
== system a20210929KillSwitchCharging/Charging ==
  AC Source : Subsystem
  AC Source1 : Subsystem  Commented=on
  Current Sensor : fl_lib/Electrical/Electrical Sensors/Current Sensor
  Current Sensor1 : fl_lib/Electrical/Electrical Sensors/Current Sensor
  DC Source : Subsystem
  Data Type Conversion{,1..3} (4 alike) : DataTypeConversion
  Electrical Reference : fl_lib/Electrical/Electrical Elements/Electrical Reference
  Electrical Reference1 : fl_lib/Electrical/Electrical Elements/Electrical Reference
  Electrical Reference3 : fl_lib/Electrical/Electrical Elements/Electrical Reference  Commented=on
  MATLAB Function : MATLAB Function  TreatAsAtomicUnit=on
  MATLAB Function1 : MATLAB Function  TreatAsAtomicUnit=on
  Open Circuit1 : fl_lib/Electrical/Electrical Elements/Open Circuit  v_specify=off  v_priority=None  v=0 V  v_nominal_specify=off  v_nominal_unit=V  v_nominal_value=1
      settings: SourceProductBaseCode=SS
  Open Circuit2 : fl_lib/Electrical/Electrical Elements/Open Circuit  v_specify=off  v_priority=None  v=0 V  v_nominal_specify=off  v_nominal_unit=V  v_nominal_value=1
      settings: SourceProductBaseCode=SS
  PS-Simulink Converter{,1..3} (4 alike) : nesl_utility/PS-Simulink Converter  PhysicalDomain=network_engine_domain  SubClassName=ps_output  LeftPortType=input  RightPortType=output  PseudoPeriodic=off  Frequencies=[]  Unit=inherit  AffineConversion=off
      settings: SourceProductBaseCode=PW,SS
  PS-Simulink Converter5 : nesl_utility/PS-Simulink Converter  Commented=on  PhysicalDomain=network_engine_domain  SubClassName=ps_output  LeftPortType=input  RightPortType=output  PseudoPeriodic=off  Frequencies=[]  Unit=inherit  AffineConversion=off
      settings: SourceProductBaseCode=PW,SS
  SPDT Switch : ee_lib/Switches & Breakers/SPDT Switch  R_closed=0.01 Ohm  G_open=1e-6 S  Threshold=0.5 V  Width=0 V  model_dynamics=0  t_on=1e-3 s  t_off=1e-3 s  initial_vT=0 V
      settings: SourceProductBaseCode=PS
  SPDT Switch1 : ee_lib/Switches & Breakers/SPDT Switch  R_closed=0.01 Ohm  G_open=1e-6 S  Threshold=0.5 V  Width=0 V  model_dynamics=0  t_on=1e-3 s  t_off=1e-3 s  initial_vT=0 V
      settings: SourceProductBaseCode=PS
  Simulink-PS Converter{,1..3} (4 alike) : nesl_utility/Simulink-PS Converter  PhysicalDomain=network_engine_domain  SubClassName=ps_input  LeftPortType=input  RightPortType=output  PseudoPeriodic=off  Frequencies=[]  NoiseDistribution=none  NoiseParameters=[]  Unit=1  AffineConversion=off  FilteringAndDerivatives=provide  SimscapeFilterOrder=1  InputFilterTimeConstant=0.001  UdotUserProvided=0
      settings: SourceProductBaseCode=PW,SS
  Solver Configuration : nesl_utility/Solver Configuration  Commented=on  PhysicalDomain=network_engine_domain  SubClassName=solver  LeftPortType=input  RightPortType=generic  Tones=[]  Harmonics=[]  SimulateNoise=off  Profile=off  UseLocalSampling=off  EnableSwitchedLinearOptims=on  FrequencyDomain=off  UseCCode=off  RelTol=0.001  AbsTol=1e-06  MinStep=1e-09  ToWorkspace=off  RevertToSquareIcSolve=off  NumHomotopyIterations=100  PhasorMode=off  PhasorModeNumHarmonics=1  DoDC=off  ResidualTolerance=1e-09  UseLocalSolver=off  LocalSolverChoice=NE_BACKWARD_EULER_ADVANCER  LocalSolverSampleTime=0.001  DoFixedCost=off  MaxNonlinIter=3  MaxModeIter=2  ComputeImpulses=off  ImpulseIterations=2  LinearAlgebra=auto  EquationFormulation=NE_TIME_EF  DelaysMemoryBudget=1024  AutomaticFiltering=on  FilteringTimeConstant=0.001  PartitionStorageMethod=AS_NEEDED  PartitionMemoryBudget=1024  PartitionMethod=ROBUST
      settings: SourceProductBaseCode=PW,SS
  Switch : fl_lib/Electrical/Electrical Elements/Switch  R_closed=0.01 Ohm  G_open=1e-8 1/Ohm  Threshold=0.5  i_specify=off  i_priority=None  i=0 A  i_nominal_specify=off  i_nominal_unit=A  i_nominal_value=1  v_specify=off  v_priority=None  v=0 V  v_nominal_specify=off  v_nominal_unit=V  v_nominal_value=1
  Switch1 : fl_lib/Electrical/Electrical Elements/Switch  R_closed=0.01 Ohm  G_open=1e-8 1/Ohm  Threshold=0.5  i_specify=off  i_priority=None  i=0 A  i_nominal_specify=off  i_nominal_unit=A  i_nominal_value=1  v_specify=off  v_priority=None  v=0 V  v_nominal_specify=off  v_nominal_unit=V  v_nominal_value=1
  Terminator : Terminator
  Terminator1 : Terminator
  Terminator3 : Terminator  Commented=on
  Voltage Sensor : fl_lib/Electrical/Electrical Sensors/Voltage Sensor
  Voltage Sensor1 : fl_lib/Electrical/Electrical Sensors/Voltage Sensor
  Voltage Sensor4 : fl_lib/Electrical/Electrical Sensors/Voltage Sensor  Commented=on
  + : PMIOPort  Side=Left
  For DC-DC : PMIOPort  Port=2  Side=Right
  tag scope: ACChargeContactorVolatge=global, DCChargeContactorVolatge=global
  wires:
  [AC_CHG_Cont] -> Data Type Conversion/1
  PS-Simulink Converter/1 -> Terminator/1  "Charge Current"
  Data Type Conversion/1 -> Simulink-PS Converter1/1
  PS-Simulink Converter1/1 -> [ACChargeContactorVolatge]  "AC_Charg_Cont_Volt"
  PS-Simulink Converter2/1 -> [DCChargeContactorVolatge]  "DC_Charg_Cont_Volt"
  [DC_CHG_Cont] -> Data Type Conversion1/1
  Data Type Conversion1/1 -> Simulink-PS Converter2/1
  PS-Simulink Converter5/1 -> Terminator3/1
  PS-Simulink Converter3/1 -> Terminator1/1
  [ChargerMode] -> MATLAB Function/1(u)
  [ChargerMode] -> MATLAB Function1/1(u)
  Data Type Conversion2/1 -> Simulink-PS Converter/1
  Data Type Conversion3/1 -> Simulink-PS Converter3/1
  MATLAB Function1/1(y) -> Data Type Conversion3/1
  MATLAB Function/1(y) -> Data Type Conversion2/1
  connections:
  Electrical Reference/LConn1 -- DC Source/RConn1
  Simulink-PS Converter1/RConn1 -- SPDT Switch/LConn1
  Current Sensor/LConn1 -- +/RConn1
  Current Sensor/RConn1 -- PS-Simulink Converter/LConn1
  SPDT Switch/LConn2 -- Current Sensor/RConn2 -- SPDT Switch1/LConn2 -- Voltage Sensor1/LConn1 -- Voltage Sensor/LConn1
  Voltage Sensor/RConn2 -- SPDT Switch/RConn2 -- Switch/LConn1 -- AC Source/LConn1
  PS-Simulink Converter1/LConn1 -- Voltage Sensor/RConn1
  Voltage Sensor1/RConn2 -- SPDT Switch1/RConn2 -- Switch1/LConn1 -- DC Source/LConn1
  PS-Simulink Converter2/LConn1 -- Voltage Sensor1/RConn1
  Simulink-PS Converter2/RConn1 -- SPDT Switch1/LConn1
  Open Circuit1/LConn1 -- SPDT Switch/RConn1
  Electrical Reference3/LConn1 -- Solver Configuration/RConn1 -- Voltage Sensor4/LConn1 -- AC Source1/RConn1
  PS-Simulink Converter5/LConn1 -- Voltage Sensor4/RConn1
  Voltage Sensor4/RConn2 -- AC Source1/LConn1
  Current Sensor1/LConn1 -- AC Source/RConn1
  Current Sensor1/RConn2 -- Electrical Reference1/LConn1
  PS-Simulink Converter3/LConn1 -- Current Sensor1/RConn1
  Open Circuit2/LConn1 -- SPDT Switch1/RConn1
  Switch/RConn2 -- Switch1/RConn2 -- For DC-DC/RConn1
  Simulink-PS Converter/RConn1 -- Switch/RConn1
  Simulink-PS Converter3/RConn1 -- Switch1/RConn1

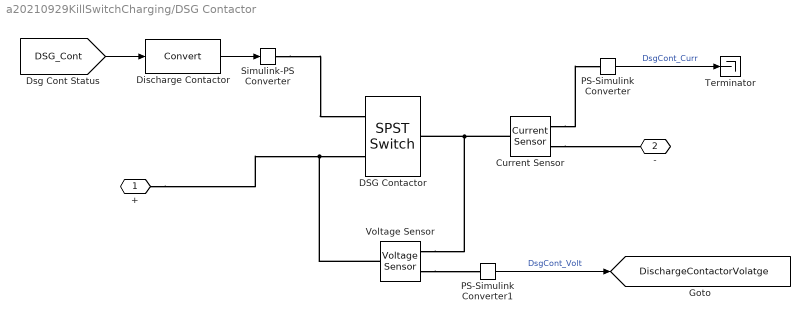
== system a20210929KillSwitchCharging/DSG Contactor ==
  Current Sensor : fl_lib/Electrical/Electrical Sensors/Current Sensor
  DSG Contactor : ee_lib/Switches & Breakers/SPST Switch  R_closed=0.01 Ohm  G_open=1e-6 S  Threshold=0.5 V  Width=0 V  model_dynamics=0  t_on=1e-3 s  t_off=1e-3 s  initial_vT=0 V
      settings: SourceProductBaseCode=PS  InternalSimscapePortConfiguration="{\"Bottom\":[],\"Left\":[{\"id\":\"vT\",\"label\":\"vT\",\"type\":\"input\"},{\"id\":\"p\",\"label\":\"\",\"type\":\"foundation.electrical.electrical\"}],\"Right\":[{\"id\":\"n\",\"label\":\"\",\"type\":\"foundation.electrical.electrical\"}],\"Top\":[]}"
  Discharge Contactor : DataTypeConversion
  PS-Simulink Converter : nesl_utility/PS-Simulink Converter  PhysicalDomain=network_engine_domain  SubClassName=ps_output  LeftPortType=input  RightPortType=output  PseudoPeriodic=off  Frequencies=[]  Unit=inherit  AffineConversion=off
      settings: SourceProductBaseCode=PW,SS
  PS-Simulink Converter1 : nesl_utility/PS-Simulink Converter  PhysicalDomain=network_engine_domain  SubClassName=ps_output  LeftPortType=input  RightPortType=output  PseudoPeriodic=off  Frequencies=[]  Unit=inherit  AffineConversion=off
      settings: SourceProductBaseCode=PW,SS
  Simulink-PS Converter : nesl_utility/Simulink-PS Converter  PhysicalDomain=network_engine_domain  SubClassName=ps_input  LeftPortType=input  RightPortType=output  PseudoPeriodic=off  Frequencies=[]  NoiseDistribution=none  NoiseParameters=[]  Unit=1  AffineConversion=off  FilteringAndDerivatives=provide  SimscapeFilterOrder=1  InputFilterTimeConstant=0.001  UdotUserProvided=0
      settings: SourceProductBaseCode=PW,SS
  Terminator : Terminator
  Voltage Sensor : fl_lib/Electrical/Electrical Sensors/Voltage Sensor
  + : PMIOPort  Side=Left
  - : PMIOPort  Port=2  Side=Right
  tag scope: DischargeContactorVolatge=global
  wires:
  PS-Simulink Converter/1 -> Terminator/1  "DsgCont_Curr"
  PS-Simulink Converter1/1 -> [DischargeContactorVolatge]  "DsgCont_Volt"
  [DSG_Cont] -> Discharge Contactor/1
  Discharge Contactor/1 -> Simulink-PS Converter/1
  connections:
  +/RConn1 -- Voltage Sensor/LConn1 -- DSG Contactor/LConn2
  Simulink-PS Converter/RConn1 -- DSG Contactor/LConn1
  Current Sensor/LConn1 -- Voltage Sensor/RConn2 -- DSG Contactor/RConn1
  Current Sensor/RConn2 -- -/RConn1
  Current Sensor/RConn1 -- PS-Simulink Converter/LConn1
  Voltage Sensor/RConn1 -- PS-Simulink Converter1/LConn1
